simulink model "CoM_2D"  (R2021b)
settings: Solver=VariableStepAuto  StartTime=0.0  StopTime=100  RelTol=1e-3
values from neighbouring files (symbols this model uses):
  g = 9.8    [simulink_test.m]
  Ixx = 0.2    [simulink_test.m]
  m = 1.0    (= 1)    [simulink_test.m]
  r = 0.11    [simulink_test.m]
  yc = 0.01    [simulink_test.m]
  zc = -0.05    [simulink_test.m]
libraries: slpidlib x3
settings Model: Creator=user  LastModifiedBy=user

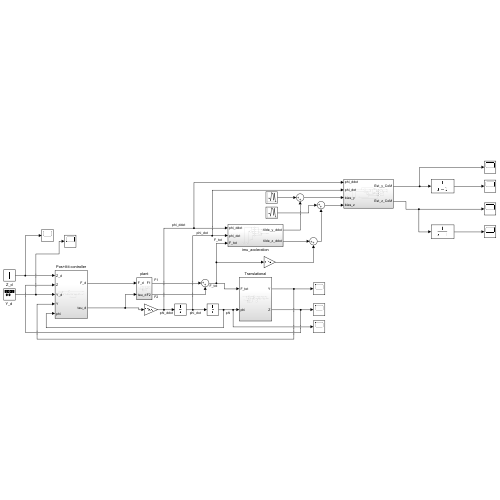
[thumbnail: Simulink's stored preview of the top-level diagram]
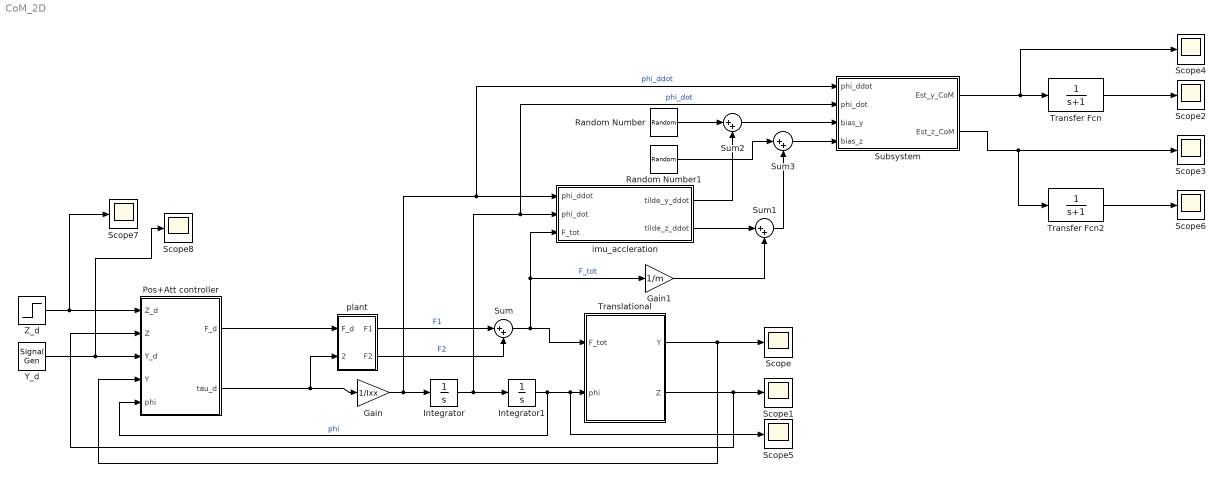
== system CoM_2D ==
  Gain : Gain  Gain=1/Ixx
  Gain1 : Gain  Gain=1/m
  Integrator : Integrator
  Integrator1 : Integrator
  Pos+Att controller : Subsystem
  Random Number : RandomNumber  SampleTime=0.005
  Random Number1 : RandomNumber  SampleTime=0.005
  Scope{,1..8} (9 alike) : Scope
  Subsystem : Subsystem
  Sum{,1..3} (4 alike) : Sum  Inputs=|++
  Transfer Fcn : TransferFcn  Denominator=[1 1]
  Transfer Fcn2 : TransferFcn  Denominator=[1 1]
  Translational : Subsystem
  "Y_d " : SignalGenerator  WaveForm=square  Frequency=0.01
  Z_d : Step  Time=0  After=-2  SampleTime=0
  imu_accleration : Subsystem
  plant : Subsystem
  wires:
  plant/1(F1) -> Sum/1  "F1"
  plant/2(F2) -> Sum/2  "F2"
  Integrator/1 -> imu_accleration/2(phi_dot), Subsystem/2(phi_dot), Integrator1/1  "phi_dot"
  Gain/1 -> imu_accleration/1(phi_ddot), Subsystem/1(phi_ddot), Integrator/1  "phi_ddot"
  Sum/1 -> Translational/1(F_tot), Gain1/1, imu_accleration/3(F_tot)  "F_tot"
  Integrator1/1 -> Pos+Att controller/5(phi), Scope5/1, Translational/2(phi)  "phi"
  Translational/1(Y) -> Pos+Att controller/4(Y), Scope/1
  Translational/2(Z) -> Pos+Att controller/2(Z), Scope1/1
  Pos+Att controller/2(tau_d) -> Gain/1, plant/2(tau_d)
  Z_d/1 -> Scope7/1, Pos+Att controller/1(Z_d)
  "Y_d "/1 -> Scope8/1, Pos+Att controller/3(Y_d)
  Pos+Att controller/1(F_d) -> plant/1(F_d)
  imu_accleration/2(tilde_z_ddot) -> Sum1/1
  Gain1/1 -> Sum1/2
  imu_accleration/1(tilde_y_ddot) -> Sum2/2
  Sum1/1 -> Sum3/2
  Subsystem/1(Est_y_CoM) -> Scope4/1, Transfer Fcn/1
  Sum2/1 -> Subsystem/3(bias_y)
  Sum3/1 -> Subsystem/4(bias_z)
  Transfer Fcn/1 -> Scope2/1
  Subsystem/2(Est_z_CoM) -> Scope3/1, Transfer Fcn2/1
  Transfer Fcn2/1 -> Scope6/1
  Random Number/1 -> Sum2/1
  Random Number1/1 -> Sum3/1

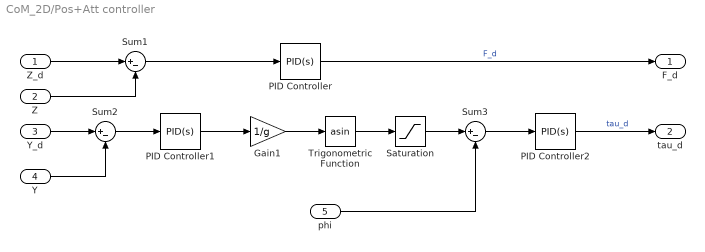
== system CoM_2D/Pos+Att controller ==
  Z_d : Inport
  Z : Inport  Port=2
  Y_d : Inport  Port=3
  Y : Inport  Port=4
  phi : Inport  Port=5
  Gain1 : Gain  Gain=1/g
  PID Controller : slpidlib/PID Controller  Controller=PID  Form=Parallel  TimeDomain=Continuous-time  UseExternalTs=off  SampleTime=-1  IntegratorMethod=Forward Euler  FilterMethod=Forward Euler  ControllerParametersSource=internal  P=20  I=3  D=15  UseFilter=on  N=100  TunerSelectOption=Transfer Function Based (PID Tuner App)  InitialConditionSource=internal  InitialConditionForIntegrator=0  InitialConditionForFilter=0  DifferentiatorICPrevScaledInput=0  ExternalReset=none  TrackingMode=off  Kt=1  LimitOutput=off  SatLimitsSource=internal  UpperSaturationLimit=inf  LowerSaturationLimit=-inf  LinearizeAsGain=on  AntiWindupMode=none  Kb=1  POutMin=[]  POutMax=[]  IOutMin=[]  IOutMax=[]  DOutMin=[]  DOutMax=[]  NOutMin=[]  NOutMax=[]  SumOutMin=[]  SumOutMax=[]  SaturationOutMin=[]  SaturationOutMax=[]  PParamMin=[]  PParamMax=[]  IParamMin=[]  IParamMax=[]  DParamMin=[]  DParamMax=[]  NParamMin=[]  NParamMax=[]  KbParamMin=[]  KbParamMax=[]  KtParamMin=[]  KtParamMax=[]  KbOutMin=[]  KbOutMax=[]  KtOutMin=[]  KtOutMax=[]  IntegratorOutMin=[]  IntegratorOutMax=[]  FilterOutMin=[]  FilterOutMax=[]  SumI1OutMin=[]  SumI1OutMax=[]  SumI2OutMin=[]  SumI2OutMax=[]  SumI3OutMin=[]  SumI3OutMax=[]  SumI4OutMin=[]  SumI4OutMax=[]  SumDOutMin=[]  SumDOutMax=[]  DifferentiatorOutMin=[]  DifferentiatorOutMax=[]  FilterDiffOutCoefMin=[]  FilterDiffOutCoefMax=[]  ReciprocalOutMin=[]  ReciprocalOutMax=[]  SumDenOutMin=[]  SumDenOutMax=[]  SumNumOutMin=[]  SumNumOutMax=[]  DivideOutMin=[]  DivideOutMax=[]  UdiffTsProdOutMin=[]  UdiffTsProdOutMax=[]  NTsProdOutMin=[]  NTsProdOutMax=[]  UintegralTsProdOutMin=[]  UintegralTsProdOutMax=[]  UngainTsProdOutMin=[]  UngainTsProdOutMax=[]  IntegratorContinuousStateAttributes=''  IntegratorStateMustResolveToSignalObject=off  IntegratorRTWStateStorageClass=Auto  FilterContinuousStateAttributes=''  FilterStateMustResolveToSignalObject=off  FilterRTWStateStorageClass=Auto  ParallelPVariant=InternalParameters  IdealPVariant=Disabled  IVariant=InternalParameters  DVariant=InternalParameters  IntegratorVariant=Continuous  SatVariant=Disabled  AWVariant=Passthrough  PCopyVariant=Disabled  TRVariant=Disabled  FdbkBlocksVariant=Forward  IdealPFdbkVariant=Disabled  SatFdbkVariant=Disabled  DerivativeFilterVariant=ContFilter  NVariant=InternalParameters  NCopyVariant=Disabled  FilterICVariant=InternalICsFilter  IntegratorICVariant=InternalICs  ExternalResetVariant=Disabled  TRSumVariant=Passthrough  SumFdbkVariant=Disabled  SumVariant=Sum_PID  TsampFilterVariant=InternalTs  TsampNgainVariant=Passthrough  TsampIntegralVariant=Passthrough  ExternalSaturationOutDataTypeStr=Inherit: Same as second input
  PID Controller1 : slpidlib/PID Controller  Controller=PID  Form=Parallel  TimeDomain=Continuous-time  UseExternalTs=off  SampleTime=-1  IntegratorMethod=Forward Euler  FilterMethod=Forward Euler  ControllerParametersSource=internal  P=2  I=0.01  D=3  UseFilter=on  N=100  TunerSelectOption=Transfer Function Based (PID Tuner App)  InitialConditionSource=internal  InitialConditionForIntegrator=0  InitialConditionForFilter=0  DifferentiatorICPrevScaledInput=0  ExternalReset=none  TrackingMode=off  Kt=1  LimitOutput=off  SatLimitsSource=internal  UpperSaturationLimit=inf  LowerSaturationLimit=-inf  LinearizeAsGain=on  AntiWindupMode=none  Kb=1  POutMin=[]  POutMax=[]  IOutMin=[]  IOutMax=[]  DOutMin=[]  DOutMax=[]  NOutMin=[]  NOutMax=[]  SumOutMin=[]  SumOutMax=[]  SaturationOutMin=[]  SaturationOutMax=[]  PParamMin=[]  PParamMax=[]  IParamMin=[]  IParamMax=[]  DParamMin=[]  DParamMax=[]  NParamMin=[]  NParamMax=[]  KbParamMin=[]  KbParamMax=[]  KtParamMin=[]  KtParamMax=[]  KbOutMin=[]  KbOutMax=[]  KtOutMin=[]  KtOutMax=[]  IntegratorOutMin=[]  IntegratorOutMax=[]  FilterOutMin=[]  FilterOutMax=[]  SumI1OutMin=[]  SumI1OutMax=[]  SumI2OutMin=[]  SumI2OutMax=[]  SumI3OutMin=[]  SumI3OutMax=[]  SumI4OutMin=[]  SumI4OutMax=[]  SumDOutMin=[]  SumDOutMax=[]  DifferentiatorOutMin=[]  DifferentiatorOutMax=[]  FilterDiffOutCoefMin=[]  FilterDiffOutCoefMax=[]  ReciprocalOutMin=[]  ReciprocalOutMax=[]  SumDenOutMin=[]  SumDenOutMax=[]  SumNumOutMin=[]  SumNumOutMax=[]  DivideOutMin=[]  DivideOutMax=[]  UdiffTsProdOutMin=[]  UdiffTsProdOutMax=[]  NTsProdOutMin=[]  NTsProdOutMax=[]  UintegralTsProdOutMin=[]  UintegralTsProdOutMax=[]  UngainTsProdOutMin=[]  UngainTsProdOutMax=[]  IntegratorContinuousStateAttributes=''  IntegratorStateMustResolveToSignalObject=off  IntegratorRTWStateStorageClass=Auto  FilterContinuousStateAttributes=''  FilterStateMustResolveToSignalObject=off  FilterRTWStateStorageClass=Auto  ParallelPVariant=InternalParameters  IdealPVariant=Disabled  IVariant=InternalParameters  DVariant=InternalParameters  IntegratorVariant=Continuous  SatVariant=Disabled  AWVariant=Passthrough  PCopyVariant=Disabled  TRVariant=Disabled  FdbkBlocksVariant=Forward  IdealPFdbkVariant=Disabled  SatFdbkVariant=Disabled  DerivativeFilterVariant=ContFilter  NVariant=InternalParameters  NCopyVariant=Disabled  FilterICVariant=InternalICsFilter  IntegratorICVariant=InternalICs  ExternalResetVariant=Disabled  TRSumVariant=Passthrough  SumFdbkVariant=Disabled  SumVariant=Sum_PID  TsampFilterVariant=InternalTs  TsampNgainVariant=Passthrough  TsampIntegralVariant=Passthrough  ExternalSaturationOutDataTypeStr=Inherit: Same as second input
  PID Controller2 : slpidlib/PID Controller  Controller=PID  Form=Parallel  TimeDomain=Continuous-time  UseExternalTs=off  SampleTime=-1  IntegratorMethod=Forward Euler  FilterMethod=Forward Euler  ControllerParametersSource=internal  P=3  I=0  D=3  UseFilter=on  N=100  TunerSelectOption=Transfer Function Based (PID Tuner App)  InitialConditionSource=internal  InitialConditionForIntegrator=0  InitialConditionForFilter=0  DifferentiatorICPrevScaledInput=0  ExternalReset=none  TrackingMode=off  Kt=1  LimitOutput=off  SatLimitsSource=internal  UpperSaturationLimit=inf  LowerSaturationLimit=-inf  LinearizeAsGain=on  AntiWindupMode=none  Kb=1  POutMin=[]  POutMax=[]  IOutMin=[]  IOutMax=[]  DOutMin=[]  DOutMax=[]  NOutMin=[]  NOutMax=[]  SumOutMin=[]  SumOutMax=[]  SaturationOutMin=[]  SaturationOutMax=[]  PParamMin=[]  PParamMax=[]  IParamMin=[]  IParamMax=[]  DParamMin=[]  DParamMax=[]  NParamMin=[]  NParamMax=[]  KbParamMin=[]  KbParamMax=[]  KtParamMin=[]  KtParamMax=[]  KbOutMin=[]  KbOutMax=[]  KtOutMin=[]  KtOutMax=[]  IntegratorOutMin=[]  IntegratorOutMax=[]  FilterOutMin=[]  FilterOutMax=[]  SumI1OutMin=[]  SumI1OutMax=[]  SumI2OutMin=[]  SumI2OutMax=[]  SumI3OutMin=[]  SumI3OutMax=[]  SumI4OutMin=[]  SumI4OutMax=[]  SumDOutMin=[]  SumDOutMax=[]  DifferentiatorOutMin=[]  DifferentiatorOutMax=[]  FilterDiffOutCoefMin=[]  FilterDiffOutCoefMax=[]  ReciprocalOutMin=[]  ReciprocalOutMax=[]  SumDenOutMin=[]  SumDenOutMax=[]  SumNumOutMin=[]  SumNumOutMax=[]  DivideOutMin=[]  DivideOutMax=[]  UdiffTsProdOutMin=[]  UdiffTsProdOutMax=[]  NTsProdOutMin=[]  NTsProdOutMax=[]  UintegralTsProdOutMin=[]  UintegralTsProdOutMax=[]  UngainTsProdOutMin=[]  UngainTsProdOutMax=[]  IntegratorContinuousStateAttributes=''  IntegratorStateMustResolveToSignalObject=off  IntegratorRTWStateStorageClass=Auto  FilterContinuousStateAttributes=''  FilterStateMustResolveToSignalObject=off  FilterRTWStateStorageClass=Auto  ParallelPVariant=InternalParameters  IdealPVariant=Disabled  IVariant=InternalParameters  DVariant=InternalParameters  IntegratorVariant=Continuous  SatVariant=Disabled  AWVariant=Passthrough  PCopyVariant=Disabled  TRVariant=Disabled  FdbkBlocksVariant=Forward  IdealPFdbkVariant=Disabled  SatFdbkVariant=Disabled  DerivativeFilterVariant=ContFilter  NVariant=InternalParameters  NCopyVariant=Disabled  FilterICVariant=InternalICsFilter  IntegratorICVariant=InternalICs  ExternalResetVariant=Disabled  TRSumVariant=Passthrough  SumFdbkVariant=Disabled  SumVariant=Sum_PID  TsampFilterVariant=InternalTs  TsampNgainVariant=Passthrough  TsampIntegralVariant=Passthrough  ExternalSaturationOutDataTypeStr=Inherit: Same as second input
  Saturation : Saturate  UpperLimit=0.3  LowerLimit=-0.3
  Sum1 : Sum  Inputs=|+-
  Sum2 : Sum  Inputs=|+-
  Sum3 : Sum  Inputs=|+-
  Trigonometric Function : Trigonometry  Operator=asin
  F_d : Outport
  tau_d : Outport  Port=2
  wires:
  Sum2/1 -> PID Controller1/1
  Sum1/1 -> PID Controller/1
  Gain1/1 -> Trigonometric Function/1
  Saturation/1 -> Sum3/1
  Sum3/1 -> PID Controller2/1
  phi/1 -> Sum3/2
  Trigonometric Function/1 -> Saturation/1
  PID Controller1/1 -> Gain1/1
  PID Controller/1 -> F_d/1  "F_d"
  Y/1 -> Sum2/2
  Z_d/1 -> Sum1/1
  PID Controller2/1 -> tau_d/1  "tau_d"
  Y_d/1 -> Sum2/1
  Z/1 -> Sum1/2

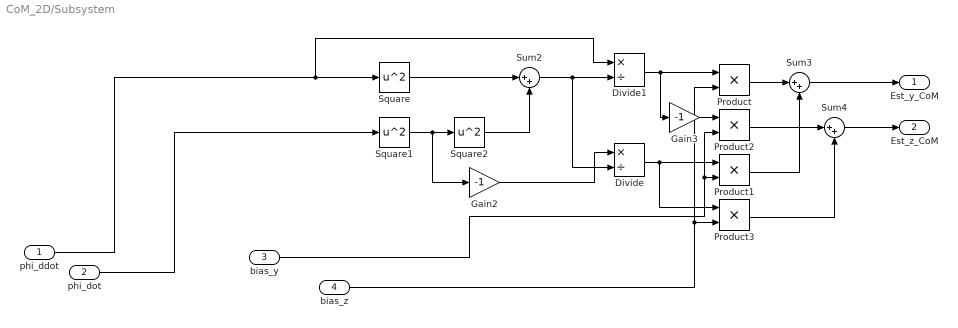
== system CoM_2D/Subsystem ==
  phi_ddot : Inport
  phi_dot : Inport  Port=2
  bias_y : Inport  Port=3
  bias_z : Inport  Port=4
  Divide : Product  Inputs=*/
  Divide1 : Product  Inputs=*/
  Gain2 : Gain  Gain=-1
  Gain3 : Gain  Gain=-1
  Product{,1..3} (4 alike) : Product
  Square : Math  Operator=square  SaturateOnIntegerOverflow=on
  Square1 : Math  Operator=square  SaturateOnIntegerOverflow=on
  Square2 : Math  Operator=square  SaturateOnIntegerOverflow=on
  Sum2 : Sum  Inputs=|++
  Sum3 : Sum  Inputs=|++
  Sum4 : Sum  Inputs=|++
  Est_y_CoM : Outport
  Est_z_CoM : Outport  Port=2
  wires:
  Divide1/1 -> Gain3/1, Product/1
  Divide/1 -> Product3/1, Product1/1
  Product1/1 -> Sum3/2
  Square2/1 -> Sum2/2
  Sum3/1 -> Est_y_CoM/1
  Square/1 -> Sum2/1
  phi_dot/1 -> Square1/1
  Sum4/1 -> Est_z_CoM/1
  bias_z/1 -> Product3/2, Product/2
  Square1/1 -> Gain2/1, Square2/1
  Gain2/1 -> Divide/1
  Product/1 -> Sum3/1
  bias_y/1 -> Product2/2, Product1/2
  Gain3/1 -> Product2/1
  Sum2/1 -> Divide1/2, Divide/2
  phi_ddot/1 -> Divide1/1, Square/1
  Product3/1 -> Sum4/2
  Product2/1 -> Sum4/1

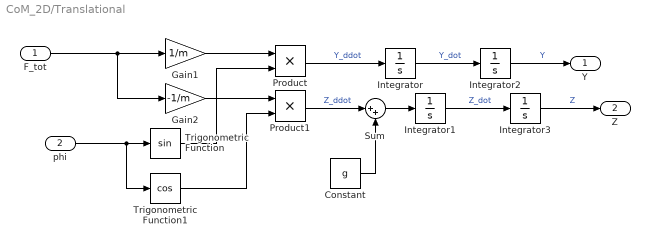
== system CoM_2D/Translational ==
  F_tot : Inport
  phi : Inport  Port=2
  Constant : Constant  Value=g
  Gain1 : Gain  Gain=1/m
  Gain2 : Gain  Gain=-1/m
  Integrator{,1..3} (4 alike) : Integrator
  Product : Product
  Product1 : Product
  Sum : Sum  Inputs=|++
  Trigonometric Function : Trigonometry
  Trigonometric Function1 : Trigonometry  Operator=cos
  Y : Outport
  Z : Outport  Port=2
  wires:
  Trigonometric Function1/1 -> Product1/2
  phi/1 -> Trigonometric Function1/1, Trigonometric Function/1
  Trigonometric Function/1 -> Product/2
  Product1/1 -> Sum/1  "Z_ddot"
  Gain2/1 -> Product1/1
  F_tot/1 -> Gain2/1, Gain1/1
  Gain1/1 -> Product/1
  Product/1 -> Integrator/1  "Y_ddot"
  Integrator/1 -> Integrator2/1  "Y_dot"
  Integrator1/1 -> Integrator3/1  "Z_dot"
  Integrator2/1 -> Y/1  "Y"
  Integrator3/1 -> Z/1  "Z"
  Sum/1 -> Integrator1/1
  Constant/1 -> Sum/2

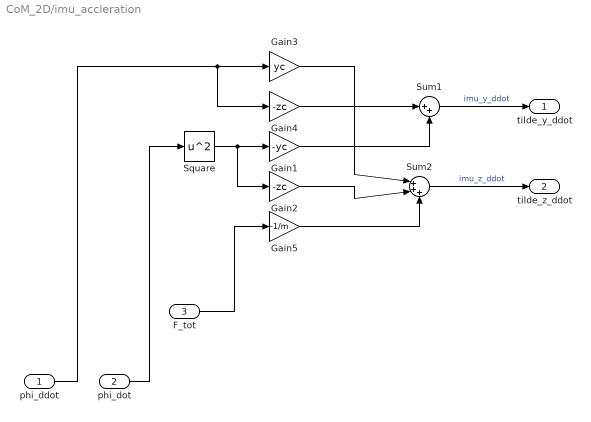
== system CoM_2D/imu_accleration ==
  phi_ddot : Inport
  phi_dot : Inport  Port=2
  F_tot : Inport  Port=3
  Gain1 : Gain  Gain=-yc
  Gain2 : Gain  Gain=-zc
  Gain3 : Gain  Gain=yc
  Gain4 : Gain  Gain=-zc
  Gain5 : Gain  Gain=-1/m
  Square : Math  Operator=square  SaturateOnIntegerOverflow=on
  Sum1 : Sum  Inputs=|++
  Sum2 : Sum  Inputs=|+++
  tilde_y_ddot : Outport
  tilde_z_ddot : Outport  Port=2
  wires:
  Gain5/1 -> Sum2/3
  Sum2/1 -> tilde_z_ddot/1  "imu_z_ddot"
  Gain4/1 -> Sum1/1
  phi_ddot/1 -> Gain4/1, Gain3/1
  Gain1/1 -> Sum1/2
  F_tot/1 -> Gain5/1
  Gain2/1 -> Sum2/2
  Gain3/1 -> Sum2/1
  Square/1 -> Gain2/1, Gain1/1
  Sum1/1 -> tilde_y_ddot/1  "imu_y_ddot"
  phi_dot/1 -> Square/1

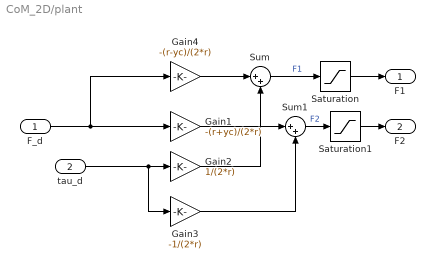
== system CoM_2D/plant ==
  F_d : Inport
  tau_d : Inport  Port=2
  Gain1 : Gain  Gain=-(r+yc)/(2*r)
  Gain2 : Gain  Gain=1/(2*r)
  Gain3 : Gain  Gain=-1/(2*r)
  Gain4 : Gain  Gain=-(r-yc)/(2*r)
  Saturation : Saturate  UpperLimit=7  LowerLimit=0
  Saturation1 : Saturate  UpperLimit=7  LowerLimit=0
  Sum : Sum  Inputs=|++
  Sum1 : Sum  Inputs=|++
  F1 : Outport
  F2 : Outport  Port=2
  wires:
  tau_d/1 -> Gain3/1, Gain2/1
  Gain2/1 -> Sum/2
  Sum/1 -> Saturation/1  "F1"
  Gain3/1 -> Sum1/2
  Sum1/1 -> Saturation1/1  "F2"
  Saturation/1 -> F1/1
  Saturation1/1 -> F2/1
  F_d/1 -> Gain4/1, Gain1/1
  Gain4/1 -> Sum/1
  Gain1/1 -> Sum1/1
